simulink model "stp1_1sym"  (R2022b)
settings: Solver=VariableStepAuto  StartTime=0.0  StopTime=10  RelTol=1e-3
settings Model: Creator=zalew  LastModifiedBy=zalew

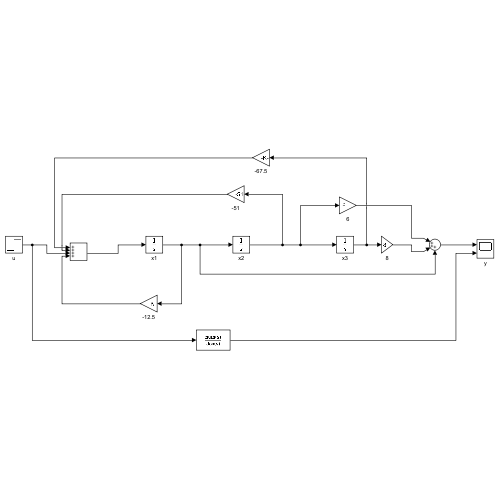
[thumbnail: Simulink's stored preview of the top-level diagram]
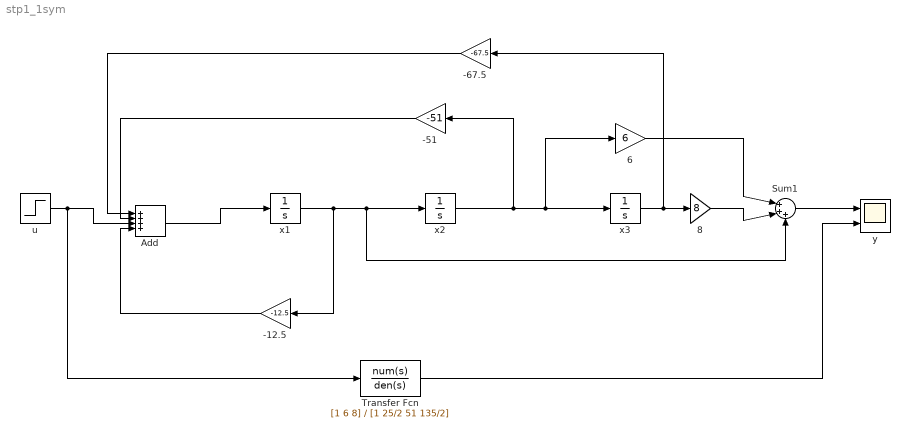
== system stp1_1sym ==
  -12.5 : Gain  Gain=-12.5
  -51 : Gain  Gain=-51
  -67.5 : Gain  Gain=-67.5
  6 : Gain  Gain=6
  8 : Gain  Gain=8
  Add : Sum  Inputs=++++
  Sum1 : Sum  Inputs=|+++
  Transfer Fcn : TransferFcn  Numerator=[1 6 8]  Denominator=[1 25/2 51 135/2]
  u : Step  After=0.4  SampleTime=0
  x1 : Integrator
  x2 : Integrator
  x3 : Integrator
  y : Scope  NumInputPorts=2
  wires:
  Add/1 -> x1/1
  x1/1 -> -12.5/1, Sum1/3, x2/1
  x2/1 -> -51/1, 6/1, x3/1
  x3/1 -> -67.5/1, 8/1
  Sum1/1 -> y/1
  -12.5/1 -> Add/4
  u/1 -> Transfer Fcn/1, Add/3
  -51/1 -> Add/2
  -67.5/1 -> Add/1
  8/1 -> Sum1/2
  6/1 -> Sum1/1
  Transfer Fcn/1 -> y/2
